simulink model "Phoenix_Main"  (R2020b)
settings: Solver=VariableStepAuto  StartTime=0.0  StopTime=10  FixedStep=0.0005  RelTol=1e-3
model workspace (MAT data in the model file):
  CL = Simulink.Parameter
  CL.Value = -3.48e-06
  CL.DataType = 'auto'
  CL.Dimensions = [1 1]
  Cm = Simulink.Parameter
  Cm.Value = -3.44e-07
  Cm.DataType = 'auto'
  Cm.Dimensions = [1 1]
  J = Simulink.Parameter
  J.Value = [0.0144  0  0; 0  0.006389  0; 0  0  0.0176]
  J.DataType = 'auto'
  J.Dimensions = [3 3]
  Motor_Rads_Max = Simulink.Parameter
  Motor_Rads_Max.Value = 800
  Motor_Rads_Max.DataType = 'auto'
  Motor_Rads_Max.Dimensions = [1 1]
  P_Att = Simulink.Parameter
  P_Att.Value = [5.3 20 3]
  P_Att.DataType = 'auto'
  P_Att.Dimensions = [1 3]
  Pos_DR = Simulink.Parameter
  Pos_DR.Value = [0.85 0.85 0.83]
  Pos_DR.DataType = 'auto'
  Pos_DR.Dimensions = [1 3]
  Pos_TC = Simulink.Parameter
  Pos_TC.Value = [0.5 0.5 0.3]
  Pos_TC.DataType = 'auto'
  Pos_TC.Dimensions = [1 3]
  Rate_Max = Simulink.Parameter
  Rate_Max.Value = [40 100 0.4]
  Rate_Max.DataType = 'auto'
  Rate_Max.Dimensions = [1 3]
  Rates_TC = Simulink.Parameter
  Rates_TC.Value = [0.05 0.085 0.044]
  Rates_TC.DataType = 'auto'
  Rates_TC.Dimensions = [1 3]
  Roll_Arm = Simulink.Parameter
  Roll_Arm.Value = 0.2
  Roll_Arm.DataType = 'auto'
  Roll_Arm.Dimensions = [1 1]
  Yaw_Arm = Simulink.Parameter
  Yaw_Arm.Value = 0.08
  Yaw_Arm.DataType = 'auto'
  Yaw_Arm.Dimensions = [1 1]
  Yaw_prop = Simulink.Parameter
  Yaw_prop.Value = 1.795e-07
  Yaw_prop.DataType = 'auto'
  Yaw_prop.Dimensions = [1 1]
  g = Simulink.Parameter
  g.Value = 9.8
  g.DataType = 'auto'
  g.Dimensions = [1 1]
  kl = Simulink.Parameter
  kl.Value = 3.48e-06
  kl.DataType = 'auto'
  kl.Dimensions = [1 1]
  km = Simulink.Parameter
  km.Value = 0.023
  km.DataType = 'auto'
  km.Dimensions = [1 1]
  kp = Simulink.Parameter
  kp.Value = 3.44e-07
  kp.DataType = 'auto'
  kp.Dimensions = [1 1]
  kt = Simulink.Parameter
  kt.Value = 7.864e-06
  kt.DataType = 'auto'
  kt.Dimensions = [1 1]
  l = Simulink.Parameter
  l.Value = 0.3
  l.DataType = 'auto'
  l.Dimensions = [1 1]
  mass = Simulink.Parameter
  mass.Value = 0.6
  mass.DataType = 'auto'
  mass.Dimensions = [1 1]
  r2t = Simulink.Parameter
  r2t.Value = 7.864e-06
  r2t.DataType = 'auto'
  r2t.Dimensions = [1 1]
libraries: sharedutil x3, sharedtransform x1, dspmathops x1, shared6dof x1
settings Model: Creator=yilun  LastModifiedBy=ruthu
settings DataIOCC: ReturnWorkspaceOutputs=off
settings DebuggingCC: ArithmeticOperatorsInVariantConditions=warning
settings SFSimCC: SimUseLocalCustomCode=off  CustomCodeUndefinedFunction=UseInterfaceOnly
settings RTWCC: RTWUseLocalCustomCode=off
settings CodeAppCC: StateflowObjectComments=on

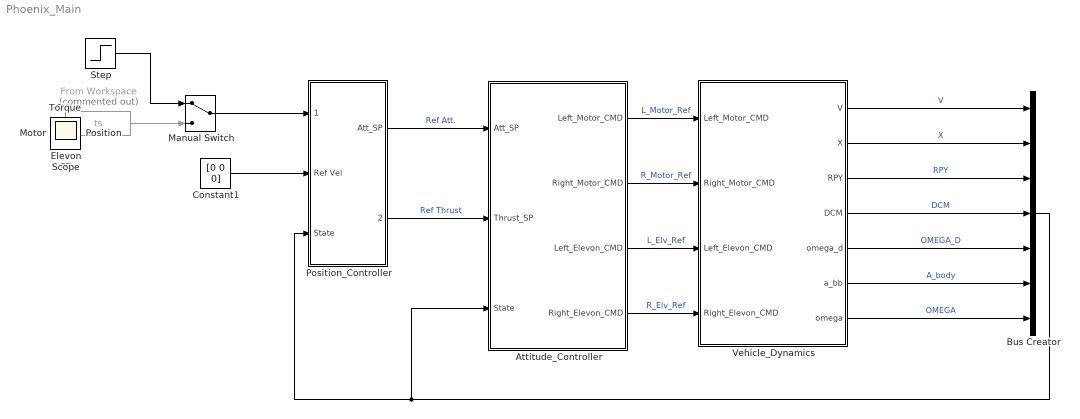
== system Phoenix_Main ==
  Attitude_Controller : Subsystem
  Bus Creator : BusCreator  Inputs=7
  Constant1 : Constant  Value=[0 0 0]
  From Workspace : FromWorkspace  Commented=on  VariableName=ts
  Manual Switch : ManualSwitch
  Position_Controller : Subsystem
  Step : Step  Time=5  Before=[0 0 -0 0]  After=[-1 0 -0 0]  SampleTime=0
  Vehicle_Dynamics : Subsystem
  Elevon : Scope
  FT : Scope
  Motor : Scope
  Position : Scope
  RPY : Scope
  Scope : Scope
  Torque : Scope
  wires:
  Position_Controller/1(Att_SP) -> Attitude_Controller/1(Att_SP)  "Ref Att."
  Vehicle_Dynamics/7(omega) -> Bus Creator/7  "OMEGA"
  Vehicle_Dynamics/1(V) -> Bus Creator/1  "V"
  Vehicle_Dynamics/2(X) -> Bus Creator/2  "X"
  Vehicle_Dynamics/3(RPY) -> Bus Creator/3  "RPY"
  Vehicle_Dynamics/4(DCM) -> Bus Creator/4  "DCM"
  Vehicle_Dynamics/5(omega_d) -> Bus Creator/5  "OMEGA_D"
  Vehicle_Dynamics/6(a_bb) -> Bus Creator/6  "A_body"
  Attitude_Controller/4(Right_Elevon_CMD) -> Vehicle_Dynamics/4(Right_Elevon_CMD)  "R_Elv_Ref"
  Attitude_Controller/3(Left_Elevon_CMD) -> Vehicle_Dynamics/3(Left_Elevon_CMD)  "L_Elv_Ref"
  Attitude_Controller/2(Right_Motor_CMD) -> Vehicle_Dynamics/2(Right_Motor_CMD)  "R_Motor_Ref"
  Attitude_Controller/1(Left_Motor_CMD) -> Vehicle_Dynamics/1(Left_Motor_CMD)  "L_Motor_Ref"
  Bus Creator/1 -> Position_Controller/3(State), Attitude_Controller/3(State)
  Position_Controller/2(Avg_Thrust_SP) -> Attitude_Controller/2(Thrust_SP)  "Ref Thrust"
  Constant1/1 -> Position_Controller/2(Ref Vel)
  Manual Switch/1 -> Position_Controller/1(Ref Pose)
  Step/1 -> Manual Switch/1
  From Workspace/1 -> Manual Switch/2

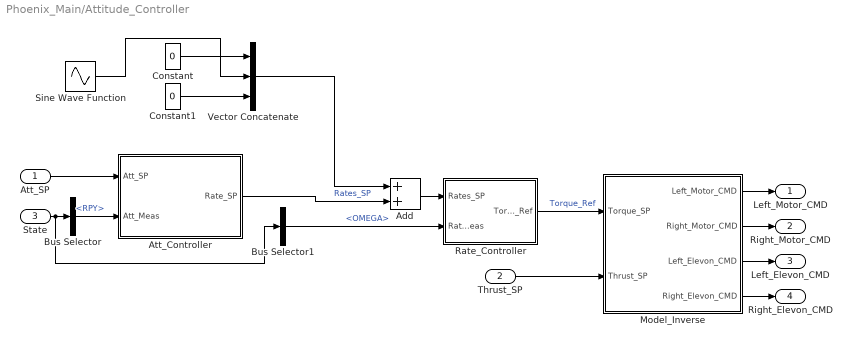
== system Phoenix_Main/Attitude_Controller ==
  Att_SP : Inport
  Thrust_SP : Inport  Port=2
  State : Inport  Port=3
  Add : Sum
  Att_Controller : Subsystem
  Bus Selector : BusSelector  OutputSignals=RPY
  Bus Selector1 : BusSelector  OutputSignals=OMEGA
  Constant : Constant  Value=0
  Constant1 : Constant  Value=0
  Model_Inverse : Subsystem
  Rate_Controller : Subsystem
  Sine Wave Function : Sin  Amplitude=0  Frequency=9.66  SampleTime=0
  Vector Concatenate : Concatenate  NumInputs=3
  Left_Motor_CMD : Outport
  Right_Motor_CMD : Outport  Port=2
  Left_Elevon_CMD : Outport  Port=3
  Right_Elevon_CMD : Outport  Port=4
  wires:
  Model_Inverse/4(Right_Elevon_CMD) -> Right_Elevon_CMD/1
  Thrust_SP/1 -> Model_Inverse/2(Thrust_SP)
  Model_Inverse/1(Left_Motor_CMD) -> Left_Motor_CMD/1
  Model_Inverse/3(Left_Elevon_CMD) -> Left_Elevon_CMD/1
  Model_Inverse/2(Right_Motor_CMD) -> Right_Motor_CMD/1
  Bus Selector1/1 -> Rate_Controller/2(Rates_Meas)  "<OMEGA>"
  Rate_Controller/1(Torque_Ref) -> Model_Inverse/1(Torque_SP)  "Torque_Ref"
  Att_Controller/1(Rate_SP) -> Add/2  "Rates_SP"
  State/1 -> Bus Selector1/1, Bus Selector/1
  Bus Selector/1 -> Att_Controller/2(Att_Meas)  "<RPY>"
  Att_SP/1 -> Att_Controller/1(Att_SP)
  Add/1 -> Rate_Controller/1(Rates_SP)
  Constant/1 -> Vector Concatenate/1
  Constant1/1 -> Vector Concatenate/3
  Sine Wave Function/1 -> Vector Concatenate/2
  Vector Concatenate/1 -> Add/1

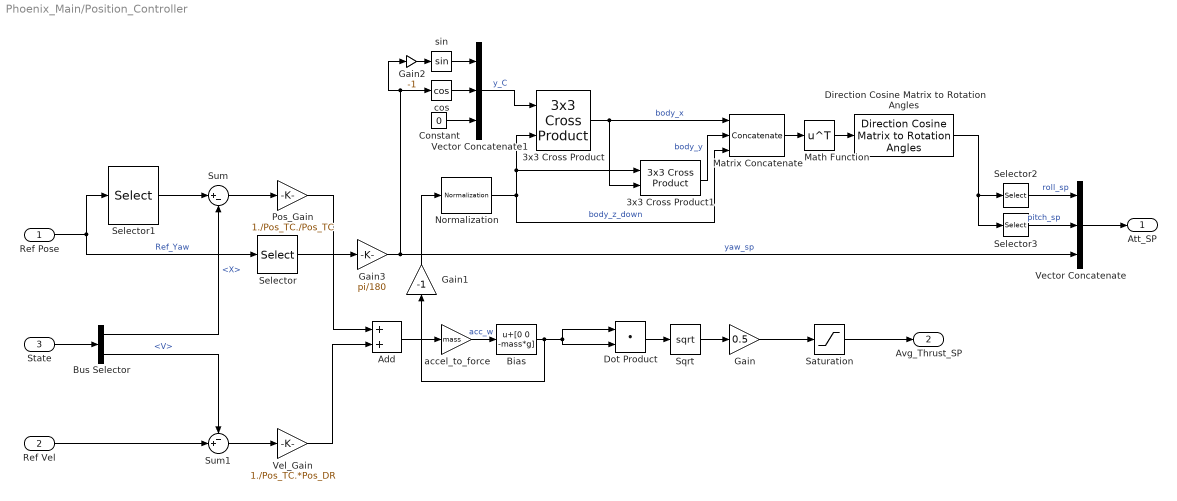
== system Phoenix_Main/Position_Controller ==
  Ref Pose : Inport
  Ref Vel : Inport  Port=2
  State : Inport  Port=3
  3x3 Cross Product : sharedutil/3x3 Cross Product  aMode=aMode
      settings: SourceProductBaseCode=AE,PW,MT,UV,VE,VP
  3x3 Cross Product1 : sharedutil/3x3 Cross Product  aMode=aMode
      settings: SourceProductBaseCode=AE,PW,MT,UV,VE,VP
  Add : Sum
  Bias : Bias  Bias=[0 0 -mass*g]
  Bus Selector : BusSelector  OutputSignals=X,V
  Constant : Constant  Value=0
  Direction Cosine Matrix to Rotation Angles : sharedtransform/Direction Cosine Matrix to Rotation Angles  rotationOrder=ZYX  aMode=aMode  action=None  tolerance=eps(2)
      settings: SourceProductBaseCode=AE,PW,MT,UV,VE,VP
  Dot Product : DotProduct  InputSameDT=on  OutDataTypeStr=Inherit: Inherit via internal rule
  Gain : Gain  Gain=0.5
  Gain1 : Gain  Gain=-1
  Gain2 : Gain  Gain=-1
  Gain3 : Gain  Gain=pi/180
  Math Function : Math  Operator=transpose  SignedPower=on  SaturateOnIntegerOverflow=on
  Matrix Concatenate : Concatenate  NumInputs=3  Mode=Multidimensional array  ConcatenateDimension=2
  Normalization : dspmathops/Normalization  NormType=2-norm  Bias=1e-10  NormOver=Each column  Dimension=1  roundingMode=Floor  overflowMode=off  accumDataTypeStr=Inherit: Same as product output  accumLastDataTypeStr=Inherit: Same as product output  outputDataTypeStr=Inherit: Same as product output  outputMin=[]  outputMax=[]  outputLastDataTypeStr=Inherit: Same as product output
  Pos_Gain : Gain  Gain=1./Pos_TC./Pos_TC
  Saturation : Saturate  UpperLimit=Inf  LowerLimit=0
  Selector : Selector  InputPortWidth=4  IndexOptions=Index vector (dialog)  Indices=4  OutputSizes=1
  Selector1 : Selector  InputPortWidth=4  IndexOptions=Index vector (dialog)  Indices=[1 2 3]  OutputSizes=1
  Selector2 : Selector  InputPortWidth=3  IndexOptions=Index vector (dialog)  Indices=3  OutputSizes=1
  Selector3 : Selector  InputPortWidth=3  IndexOptions=Index vector (dialog)  Indices=2  OutputSizes=1
  Sqrt : Sqrt  SaturateOnIntegerOverflow=on
  Sum : Sum  Inputs=|+-
  Sum1 : Sum  Inputs=-+|
  Vector Concatenate : Concatenate  NumInputs=3
  Vector Concatenate1 : Concatenate  NumInputs=3
  Vel_Gain : Gain  Gain=1./Pos_TC.*Pos_DR
  accel_to_force : Gain  Gain=mass
  cos : Trigonometry  Operator=cos
  sin : Trigonometry
  Att_SP : Outport
  Avg_Thrust_SP : Outport  Port=2
  wires:
  Vector Concatenate/1 -> Att_SP/1
  Ref Pose/1 -> Selector1/1, Selector/1  "Ref_Yaw"
  Selector/1 -> Gain3/1
  State/1 -> Bus Selector/1
  Selector1/1 -> Sum/1
  Bus Selector/1 -> Sum/2  "<X>"
  Ref Vel/1 -> Sum1/2
  Bus Selector/2 -> Sum1/1  "<V>"
  Sum/1 -> Pos_Gain/1
  Sum1/1 -> Vel_Gain/1
  Pos_Gain/1 -> Add/1
  Vel_Gain/1 -> Add/2
  Add/1 -> accel_to_force/1
  accel_to_force/1 -> Bias/1  "acc_w"
  Sqrt/1 -> Gain/1
  Bias/1 -> Dot Product/2, Dot Product/1, Gain1/1
  Gain/1 -> Saturation/1
  sin/1 -> Vector Concatenate1/1
  cos/1 -> Vector Concatenate1/2
  Constant/1 -> Vector Concatenate1/3
  Vector Concatenate1/1 -> 3x3 Cross Product/1  "y_C"
  Normalization/1 -> 3x3 Cross Product1/1, 3x3 Cross Product/2, Matrix Concatenate/3  "body_z_down"
  3x3 Cross Product/1 -> 3x3 Cross Product1/2, Matrix Concatenate/1  "body_x"
  3x3 Cross Product1/1 -> Matrix Concatenate/2  "body_y"
  Direction Cosine Matrix to Rotation Angles/1 -> Selector3/1, Selector2/1
  Selector3/1 -> Vector Concatenate/2  "pitch_sp"
  Selector2/1 -> Vector Concatenate/1  "roll_sp"
  Dot Product/1 -> Sqrt/1
  Saturation/1 -> Avg_Thrust_SP/1
  Gain1/1 -> Normalization/1
  Matrix Concatenate/1 -> Math Function/1
  Math Function/1 -> Direction Cosine Matrix to Rotation Angles/1
  Gain3/1 -> Vector Concatenate/3, Gain2/1, cos/1  "yaw_sp"
  Gain2/1 -> sin/1

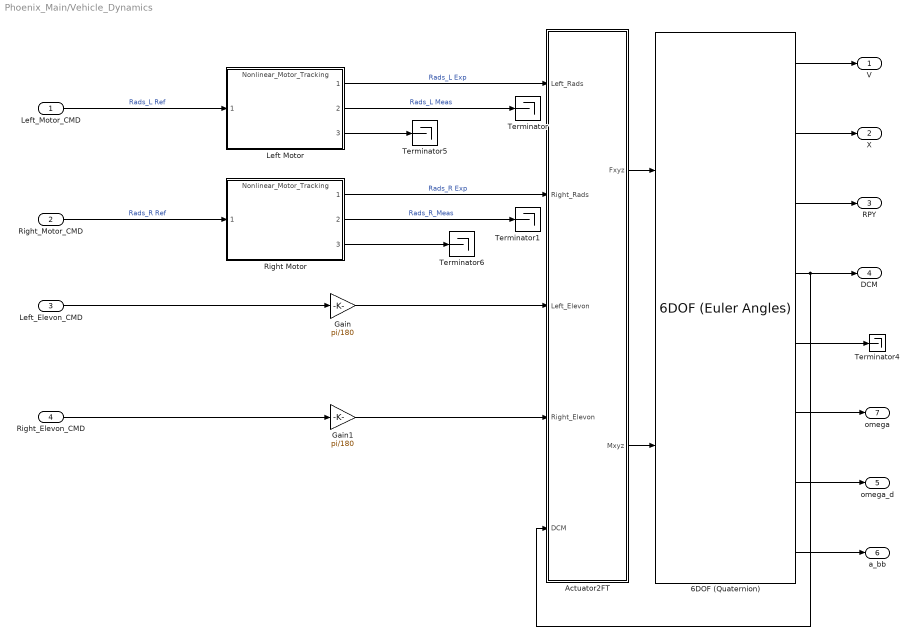
== system Phoenix_Main/Vehicle_Dynamics ==
  Left_Motor_CMD : Inport
  Right_Motor_CMD : Inport  Port=2
  Left_Elevon_CMD : Inport  Port=3
  Right_Elevon_CMD : Inport  Port=4
  6DOF (Quaternion) : shared6dof/6DOF (Euler Angles)  units=Metric (MKS)  mtype=Fixed  rep=Quaternion  xme_0=[0 0 0]  Vm_0=[0 0 0]  eul_0=[0 0 0]  pm_0=[0 0 0]  mass_0=mass  mass_e=0.5  mass_f=2.0  inertia=J  inertia_e=eye(3)  inertia_f=2*eye(3)  k_quat=1.0  vre_flag=on  abi_flag=off  aMode=aMode  xme_statename=''  Vm_statename=''  eul_statename=''  quat_statename=''  pm_statename=''  mass_statename=''
      settings: SourceProductBaseCode=AE,PW,MT,UV,VE,VP
  Actuator2FT : Subsystem
  Gain : Gain  Gain=pi/180
  Gain1 : Gain  Gain=pi/180
  Left Motor : ModelReference  ModelNameDialog=Nonlinear_Motor_Tracking.slx  ModelReferenceVersion=1.31
  Right Motor : ModelReference  ModelNameDialog=Nonlinear_Motor_Tracking.slx  ModelReferenceVersion=1.31
  Terminator{,1,4..6} (5 alike) : Terminator
  V : Outport
  X : Outport  Port=2
  RPY : Outport  Port=3
  DCM : Outport  Port=4
  omega_d : Outport  Port=5
  a_bb : Outport  Port=6
  omega : Outport  Port=7
  wires:
  6DOF (Quaternion)/6 -> omega/1
  6DOF (Quaternion)/3 -> RPY/1
  6DOF (Quaternion)/4 -> DCM/1, Actuator2FT/5(DCM)
  6DOF (Quaternion)/5 -> Terminator4/1
  6DOF (Quaternion)/8 -> a_bb/1
  6DOF (Quaternion)/1 -> V/1
  6DOF (Quaternion)/2 -> X/1
  6DOF (Quaternion)/7 -> omega_d/1
  Left_Motor_CMD/1 -> Left Motor/1  "Rads_L Ref"
  Left Motor/1 -> Actuator2FT/1(Left_Rads)  "Rads_L Exp"
  Right_Motor_CMD/1 -> Right Motor/1  "Rads_R Ref"
  Actuator2FT/1(Fxyz) -> 6DOF (Quaternion)/1
  Actuator2FT/2(Mxyz) -> 6DOF (Quaternion)/2
  Right Motor/1 -> Actuator2FT/2(Right_Rads)  "Rads_R Exp"
  Left Motor/2 -> Terminator/1  "Rads_L Meas"
  Right Motor/2 -> Terminator1/1  "Rads_R_Meas"
  Left Motor/3 -> Terminator5/1
  Right Motor/3 -> Terminator6/1
  Left_Elevon_CMD/1 -> Gain/1
  Right_Elevon_CMD/1 -> Gain1/1
  Gain/1 -> Actuator2FT/3(Left_Elevon)
  Gain1/1 -> Actuator2FT/4(Right_Elevon)

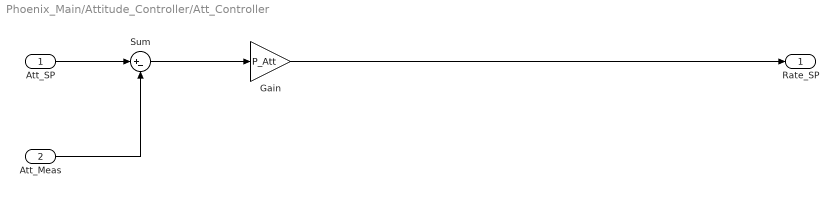
== system Phoenix_Main/Attitude_Controller/Att_Controller ==
  Att_SP : Inport
  Att_Meas : Inport  Port=2
  Gain : Gain  Gain=P_Att
  Sum : Sum  Inputs=|+-
  Rate_SP : Outport
  wires:
  Att_SP/1 -> Sum/1
  Att_Meas/1 -> Sum/2
  Sum/1 -> Gain/1
  Gain/1 -> Rate_SP/1

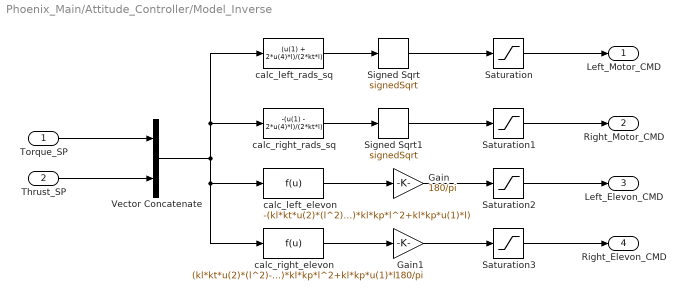
== system Phoenix_Main/Attitude_Controller/Model_Inverse ==
  Torque_SP : Inport
  Thrust_SP : Inport  Port=2
  Gain : Gain  Gain=180/pi
  Gain1 : Gain  Gain=180/pi
  Saturation : Saturate  UpperLimit=Motor_Rads_Max  LowerLimit=0
  Saturation1 : Saturate  UpperLimit=Motor_Rads_Max  LowerLimit=0
  Saturation2 : Saturate  UpperLimit=60  LowerLimit=-60
  Saturation3 : Saturate  UpperLimit=60  LowerLimit=-60
  Signed Sqrt : Sqrt  Operator=signedSqrt  SaturateOnIntegerOverflow=on
  Signed Sqrt1 : Sqrt  Operator=signedSqrt  SaturateOnIntegerOverflow=on
  Vector Concatenate : Concatenate
  calc_left_elevon : Fcn  Expr=-(kl*kt*u(2)*(l^2)+kp*kt*u(3)*l-km*kp*kt*u(1))/(2*u(4)*kl*kp*l^2+kl*kp*u(1)*l)
  calc_left_rads_sq : Fcn  Expr=(u(1) + 2*u(4)*l)/(2*kt*l)
  calc_right_elevon : Fcn  Expr=(kl*kt*u(2)*(l^2)-kp*kt*u(3)*l+km*kp*kt*u(1))/(-2*u(4)*kl*kp*l^2+kl*kp*u(1)*l)
  calc_right_rads_sq : Fcn  Expr=-(u(1) - 2*u(4)*l)/(2*kt*l)
  Left_Motor_CMD : Outport
  Right_Motor_CMD : Outport  Port=2
  Left_Elevon_CMD : Outport  Port=3
  Right_Elevon_CMD : Outport  Port=4
  wires:
  Vector Concatenate/1 -> calc_right_elevon/1, calc_left_elevon/1, calc_right_rads_sq/1, calc_left_rads_sq/1
  Thrust_SP/1 -> Vector Concatenate/2
  Torque_SP/1 -> Vector Concatenate/1
  calc_left_rads_sq/1 -> Signed Sqrt/1
  Signed Sqrt/1 -> Saturation/1
  Saturation/1 -> Left_Motor_CMD/1
  Signed Sqrt1/1 -> Saturation1/1
  Saturation1/1 -> Right_Motor_CMD/1
  calc_right_rads_sq/1 -> Signed Sqrt1/1
  calc_left_elevon/1 -> Gain/1
  Saturation2/1 -> Left_Elevon_CMD/1
  calc_right_elevon/1 -> Gain1/1
  Saturation3/1 -> Right_Elevon_CMD/1
  Gain/1 -> Saturation2/1
  Gain1/1 -> Saturation3/1

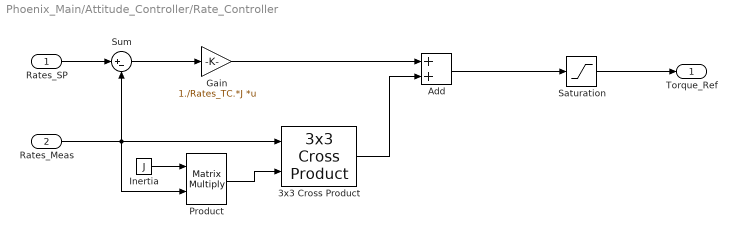
== system Phoenix_Main/Attitude_Controller/Rate_Controller ==
  Rates_SP : Inport
  Rates_Meas : Inport  Port=2
  3x3 Cross Product : sharedutil/3x3 Cross Product  aMode=aMode
      settings: SourceProductBaseCode=AE,PW,MT,UV,VE,VP
  Add : Sum
  Gain : Gain  Gain=1./Rates_TC.*J  Multiplication=Matrix(K*u)
  Inertia : Constant  Value=J
  Product : Product  Multiplication=Matrix(*)
  Saturation : Saturate  UpperLimit=Rate_Max  LowerLimit=-Rate_Max
  Sum : Sum  Inputs=|+-
  Torque_Ref : Outport
  wires:
  Rates_SP/1 -> Sum/1
  Rates_Meas/1 -> Product/2, 3x3 Cross Product/1, Sum/2
  Sum/1 -> Gain/1
  Product/1 -> 3x3 Cross Product/2
  Inertia/1 -> Product/1
  Add/1 -> Saturation/1
  Gain/1 -> Add/1
  3x3 Cross Product/1 -> Add/2
  Saturation/1 -> Torque_Ref/1

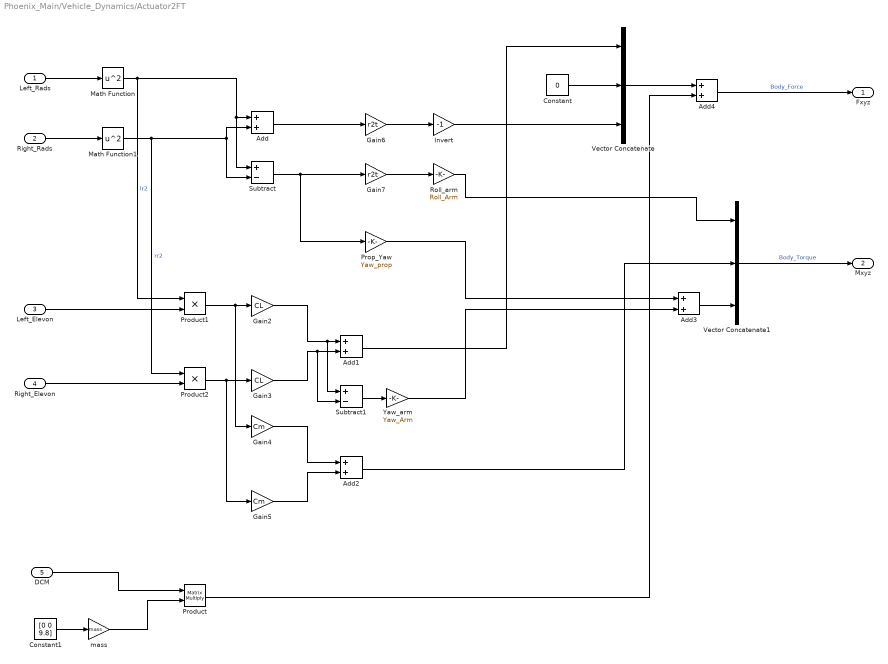
== system Phoenix_Main/Vehicle_Dynamics/Actuator2FT ==
  Left_Rads : Inport
  Right_Rads : Inport  Port=2
  Left_Elevon : Inport  Port=3
  Right_Elevon : Inport  Port=4
  DCM : Inport  Port=5
  Add{,1..4} (5 alike) : Sum
  Constant : Constant  Value=0
  Constant1 : Constant  Value=[0 0 9.8]
  Gain2 : Gain  Gain=CL
  Gain3 : Gain  Gain=CL
  Gain4 : Gain  Gain=Cm
  Gain5 : Gain  Gain=Cm
  Gain6 : Gain  Gain=r2t
  Gain7 : Gain  Gain=r2t
  Invert : Gain  Gain=-1
  Math Function : Math  Operator=square  SignedPower=on  SaturateOnIntegerOverflow=on
  Math Function1 : Math  Operator=square  SignedPower=on  SaturateOnIntegerOverflow=on
  Product : Product  Multiplication=Matrix(*)
  Product1 : Product
  Product2 : Product
  Prop_Yaw : Gain  Gain=Yaw_prop
  Roll_arm : Gain  Gain=Roll_Arm
  Subtract : Sum  Inputs=+-
  Subtract1 : Sum  Inputs=+-
  Vector Concatenate : Concatenate  NumInputs=3
  Vector Concatenate1 : Concatenate  NumInputs=3
  Yaw_arm : Gain  Gain=Yaw_Arm
  mass : Gain  Gain=mass
  Fxyz : Outport
  Mxyz : Outport  Port=2
  wires:
  Left_Rads/1 -> Math Function/1
  Right_Rads/1 -> Math Function1/1
  Math Function/1 -> Subtract/1, Add/1, Product1/1  "lr2"
  Math Function1/1 -> Add/2, Subtract/2, Product2/1  "rr2"
  Add/1 -> Gain6/1
  Invert/1 -> Vector Concatenate/3
  Constant/1 -> Vector Concatenate/2
  Add4/1 -> Fxyz/1  "Body_Force"
  Left_Elevon/1 -> Product1/2
  Product1/1 -> Gain4/1, Gain2/1
  Product2/1 -> Gain5/1, Gain3/1
  Right_Elevon/1 -> Product2/2
  Gain2/1 -> Subtract1/1, Add1/1
  Gain3/1 -> Subtract1/2, Add1/2
  Add1/1 -> Vector Concatenate/1
  Vector Concatenate1/1 -> Mxyz/1  "Body_Torque"
  Subtract/1 -> Prop_Yaw/1, Gain7/1
  Roll_arm/1 -> Vector Concatenate1/1
  Gain4/1 -> Add2/1
  Gain5/1 -> Add2/2
  Add2/1 -> Vector Concatenate1/2
  Subtract1/1 -> Yaw_arm/1
  Gain6/1 -> Invert/1
  Gain7/1 -> Roll_arm/1
  Prop_Yaw/1 -> Add3/1
  Add3/1 -> Vector Concatenate1/3
  Yaw_arm/1 -> Add3/2
  Constant1/1 -> mass/1
  DCM/1 -> Product/1
  mass/1 -> Product/2
  Vector Concatenate/1 -> Add4/1
  Product/1 -> Add4/2
